simulink library "lpr"  (Simulink 8.1)
settings: Solver=ode1  StartTime=0.0  StopTime=Inf  FixedStep=0.001  RelTol=1e-3
PostLoadFcn:
  | , if any(exist('dsrtsu_mdlpostloadfcn', 'file') == [2, 3, 6]), try dsrtsu_mdlpostloadfcn('Execute', bdroot); catch fprintf('Error in PostLoadFcn (dsrtsu_mdlpostloadfcn) for model "%s":\n %s\n', bdroot, lasterr); end, end,
undefined symbols (not defined in the file or in its folder): ENUM_LANEQUALITY_MEDIUM, FALSE, KAPP_VehicleWidth_m, KPER_C0CrossingThr_m, KPER_CalDefaultTLC_s, KPER_CalTLCMax_s, KPER_CalTLCMin_s, KPER_DefaultLaneWidth_m, KPER_LaneWidHoldOnTime_s, KPER_LaneWidRampFinErrThres_m, KPER_LaneWidRampFinTimeThres_s, KPER_LaneWidRampInFalRt_mps, KPER_LaneWidRampInRisRt_mps, KPER_LaneWidRampOutFalRt_mps, KPER_LaneWidRampOutRisRt_mps, KPER_TLCDefaultValue_s, KPER_UseCalTLC_flg, TRUE
libraries: hcu_lib x6
settings Model: DSRTSU_INTERNAL_RTI_VER=450  DSRTSU_INTERNAL_RTI_TYPE=rti1401  RTICANMMDATA=struct('GeneralSetupData',struct('modelroot','D:\ELN150201_TAIWAN\trunk\AdasDragon\software\sw_development\arch\app\per','generalsettings',struct('filesettings',struct('destfolder',struct('Name','RTICANMM_FILES','Check',1),'buildfolder',struct('Name','.','Check',1),'AbsDestfolder',struct('Name','D:\ELN150201_TAIWAN\trunk\AdasDragon\software\sw_development\arch\app\per\RTICANMM_FILES'),'AbsBuildfolder',struct('Name','D:\ELN150201_TAIWAN\trunk\AdasDragon\software\sw_development\arch\app\per'))),'options',struct('addpaths',1,'rmpaths',1,'addtrcexclusion',logical(1),'cannavigator',struct('checkmonitoring',0),'show_usrtrc',0,'use_usrtrc',0),'advanced',struct('options',[1 1 1 1 1 1 1 1 1 1 1 1 1 1 1 1 1 1 1 1 1 1 1 1 1 1 1 1 1 1 1 1 1 1 1 1 1 1 1 1 1 1 1 1 1 1 1 1 1 1 1 1 1 1 1 1 1 1 1 1 1 1 1 1 1 1 1 1 1 1 1 1 1 1 1 1 1 1 1 1 1 1 1 1 1 1 1 1 1 1 1 1 1 1 1 1 1 1 1 1]),'MPSetup',{{}},'modelname','lpr','block','lpr'))  DSRTSU_INTERNAL_RTIFPGA=40  Creator=tescamilla  LastModifiedBy=AT015555

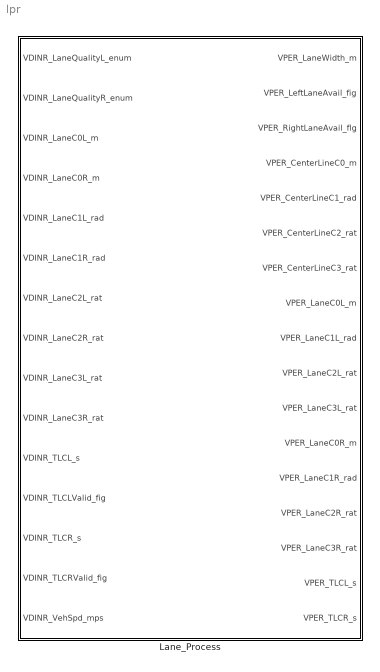
== system lpr ==
  Lane_Process : Subsystem  TreatAsAtomicUnit=on

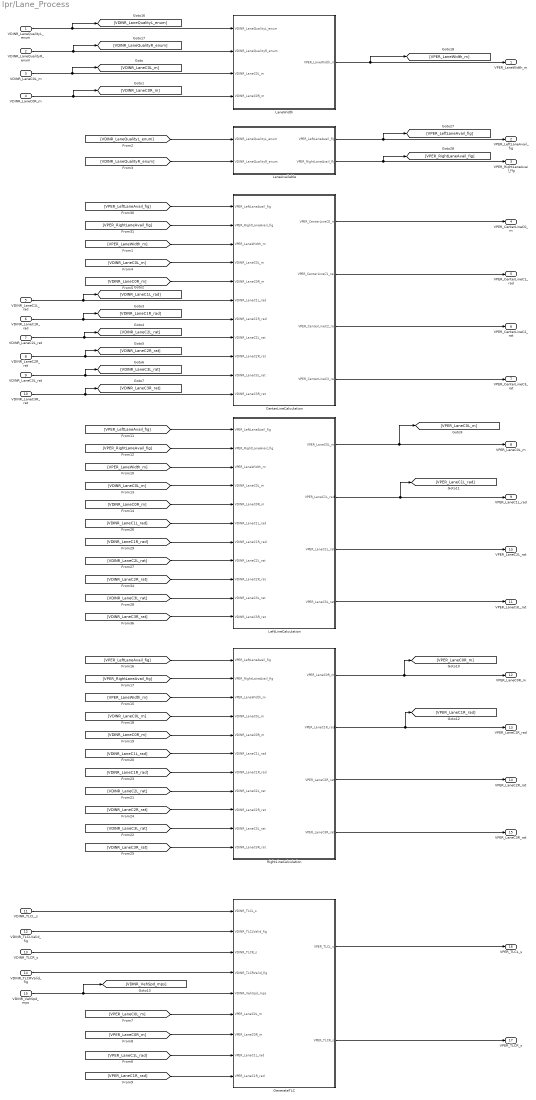
== system lpr/Lane_Process ==
  VDINR_LaneQualityL_enum : Inport
  VDINR_LaneQualityR_enum : Inport  Port=2
  VDINR_LaneC0L_m : Inport  Port=3
  VDINR_LaneC0R_m : Inport  Port=4
  VDINR_LaneC1L_rad : Inport  Port=5
  VDINR_LaneC1R_rad : Inport  Port=6
  VDINR_LaneC2L_rat : Inport  Port=7
  VDINR_LaneC2R_rat : Inport  Port=8
  VDINR_LaneC3L_rat : Inport  Port=9
  VDINR_LaneC3R_rat : Inport  Port=10
  VDINR_TLCL_s : Inport  Port=11
  VDINR_TLCLValid_fig : Inport  Port=12
  VDINR_TLCR_s : Inport  Port=13
  VDINR_TLCRValid_fig : Inport  Port=14
  VDINR_VehSpd_mps : Inport  Port=15
  CenterLineCalculation : Subsystem
  GenerateTLC : Subsystem
  LaneAvailable : Subsystem
  LaneWidth : Subsystem
  LeftLineCalculation : Subsystem
  RightLineCalculation : Subsystem
  VPER_LaneWidth_m : Outport
  VPER_LeftLaneAvail_fig : Outport  Port=2
  VPER_RightLaneAvail_flg : Outport  Port=3
  "VPER_CenterLineC0_m " : Outport  Port=4
  VPER_CenterLineC1_rad : Outport  Port=5
  VPER_CenterLineC2_rat : Outport  Port=6
  VPER_CenterLineC3_rat : Outport  Port=7
  VPER_LaneC0L_m : Outport  Port=8
  VPER_LaneC1L_rad : Outport  Port=9
  VPER_LaneC2L_rat : Outport  Port=10
  VPER_LaneC3L_rat : Outport  Port=11
  VPER_LaneC0R_m : Outport  Port=12
  VPER_LaneC1R_rad : Outport  Port=13
  VPER_LaneC2R_rat : Outport  Port=14
  VPER_LaneC3R_rat : Outport  Port=15
  VPER_TLCL_s : Outport  Port=16
  VPER_TLCR_s : Outport  Port=17
  wires:
  VDINR_LaneC1L_rad/1 -> CenterLineCalculation/6(VDINR_LaneC1L_rad), [VDINR_LaneC1L_rad]
  VDINR_LaneC1R_rad/1 -> CenterLineCalculation/7(VDINR_LaneC1R_rad), [VDINR_LaneC1R_rad]
  VDINR_LaneC2L_rat/1 -> CenterLineCalculation/8(VDINR_LaneC2L_rat), [VDINR_LaneC2L_rat]
  VDINR_LaneC2R_rat/1 -> CenterLineCalculation/9(VDINR_LaneC2R_rat), [VDINR_LaneC2R_rat]
  VDINR_LaneC3L_rat/1 -> CenterLineCalculation/10(VDINR_LaneC3L_rat), [VDINR_LaneC3L_rat]
  VDINR_LaneC3R_rat/1 -> CenterLineCalculation/11(VDINR_LaneC3R_rat), [VDINR_LaneC3R_rat]
  VDINR_LaneQualityL_enum/1 -> [VDINR_LaneQualityL_enum], LaneWidth/1(VDINR_LaneQualityL_enum)
  VDINR_LaneQualityR_enum/1 -> [VDINR_LaneQualityR_enum], LaneWidth/2(VDINR_LaneQualityR_enum)
  VDINR_LaneC0L_m/1 -> [VDINR_LaneC0L_m], LaneWidth/3(VDINR_LaneC0L_m)
  VDINR_LaneC0R_m/1 -> [VDINR_LaneC0R_m], LaneWidth/4(VDINR_LaneC0R_m)
  LaneWidth/1(VPER_LaneWidth_m) -> VPER_LaneWidth_m/1, [VPER_LaneWidth_m]
  LaneAvailable/2(VPER_RightLaneAvail_flg) -> [VPER_RightLaneAvail_fig], VPER_RightLaneAvail_flg/1
  LaneAvailable/1(VPER_LeftLaneAvail_flg) -> [VPER_LeftLaneAvail_fig], VPER_LeftLaneAvail_fig/1
  [VDINR_LaneQualityL_enum] -> LaneAvailable/1(VDINR_LaneQualityL_enum)
  [VDINR_LaneQualityR_enum] -> LaneAvailable/2(VDINR_LaneQualityR_enum)
  [VPER_LeftLaneAvail_fig] -> CenterLineCalculation/1(VPER_LeftLaneAvail_fig)
  [VPER_RightLaneAvail_fig] -> CenterLineCalculation/2(VPER_RightLaneAvail_fig)
  CenterLineCalculation/1("VPER_CenterLineC0_m ") -> "VPER_CenterLineC0_m "/1
  CenterLineCalculation/2(VPER_CenterLineC1_rad) -> VPER_CenterLineC1_rad/1
  CenterLineCalculation/3(VPER_CenterLineC2_rat) -> VPER_CenterLineC2_rat/1
  CenterLineCalculation/4(VPER_CenterLineC3_rat) -> VPER_CenterLineC3_rat/1
  VDINR_TLCL_s/1 -> GenerateTLC/1(VDINR_TLCL_s)
  VDINR_TLCLValid_fig/1 -> GenerateTLC/2(VDINR_TLCLValid_fig)
  VDINR_TLCR_s/1 -> GenerateTLC/3(VDINR_TLCR_s)
  VDINR_TLCRValid_fig/1 -> GenerateTLC/4(VDINR_TLCRValid_fig)
  GenerateTLC/1(VPER_TLCL_s) -> VPER_TLCL_s/1
  GenerateTLC/2(VPER_TLCR_s) -> VPER_TLCR_s/1
  [VPER_LaneWidth_m] -> CenterLineCalculation/3(VPER_LaneWidth_m)
  [VDINR_LaneC0L_m] -> CenterLineCalculation/4(VDINR_LaneC0L_m)
  [VDINR_LaneC0R_m] -> CenterLineCalculation/5(VDINR_LaneC0R_m)
  [VPER_LaneC1L_rad] -> GenerateTLC/8(VPER_LaneC1L_rad)
  [VPER_LaneC0L_m] -> GenerateTLC/6(VPER_LaneC0L_m)
  [VPER_LaneC0R_m] -> GenerateTLC/7(VPER_LaneC0R_m)
  VDINR_VehSpd_mps/1 -> [VDINR_VehSpd_mps], GenerateTLC/5(VDINR_VehSpd_mps)
  [VPER_LaneC1R_rad] -> GenerateTLC/9(VPER_LaneC1R_rad)
  [VDINR_LaneC0L_m] -> LeftLineCalculation/4(VDINR_LaneC0L_m)
  [VDINR_LaneC0R_m] -> LeftLineCalculation/5(VDINR_LaneC0R_m)
  [VPER_LaneWidth_m] -> LeftLineCalculation/3(VPER_LaneWidth_m)
  [VPER_RightLaneAvail_fig] -> LeftLineCalculation/2(VPER_RightLaneAvail_fig)
  [VPER_LeftLaneAvail_fig] -> LeftLineCalculation/1(VPER_LeftLaneAvail_fig)
  [VDINR_LaneC0L_m] -> RightLineCalculation/4(VDINR_LaneC0L_m)
  [VDINR_LaneC0R_m] -> RightLineCalculation/5(VDINR_LaneC0R_m)
  [VPER_LaneWidth_m] -> RightLineCalculation/3(VPER_LaneWidth_m)
  [VPER_RightLaneAvail_fig] -> RightLineCalculation/2(VPER_RightLaneAvail_fig)
  [VPER_LeftLaneAvail_fig] -> RightLineCalculation/1(VPER_LeftLaneAvail_fig)
  [VDINR_LaneC1L_rad] -> RightLineCalculation/6(VDINR_LaneC1L_rad)
  [VDINR_LaneC2L_rat] -> RightLineCalculation/8(VDINR_LaneC2L_rat)
  [VDINR_LaneC3L_rat] -> RightLineCalculation/10(VDINR_LaneC3L_rat)
  [VDINR_LaneC2R_rat] -> RightLineCalculation/9(VDINR_LaneC2R_rat)
  [VDINR_LaneC3R_rat] -> RightLineCalculation/11(VDINR_LaneC3R_rat)
  [VDINR_LaneC1R_rad] -> RightLineCalculation/7(VDINR_LaneC1R_rad)
  [VDINR_LaneC2L_rat] -> LeftLineCalculation/8(VDINR_LaneC2L_rat)
  [VDINR_LaneC2R_rat] -> LeftLineCalculation/9(VDINR_LaneC2R_rat)
  [VDINR_LaneC1L_rad] -> LeftLineCalculation/6(VDINR_LaneC1L_rad)
  [VDINR_LaneC3R_rat] -> LeftLineCalculation/11(VDINR_LaneC3R_rat)
  [VDINR_LaneC3L_rat] -> LeftLineCalculation/10(VDINR_LaneC3L_rat)
  [VDINR_LaneC1R_rad] -> LeftLineCalculation/7(VDINR_LaneC1R_rad)
  LeftLineCalculation/1(VPER_LaneC0L_m) -> VPER_LaneC0L_m/1, [VPER_LaneC0L_m]
  LeftLineCalculation/2(VPER_LaneC1L_rad) -> VPER_LaneC1L_rad/1, [VPER_LaneC1L_rad]
  LeftLineCalculation/3(VPER_LaneC2L_rat) -> VPER_LaneC2L_rat/1
  LeftLineCalculation/4(VPER_LaneC3L_rat) -> VPER_LaneC3L_rat/1
  RightLineCalculation/1(VPER_LaneC0R_m) -> VPER_LaneC0R_m/1, [VPER_LaneC0R_m]
  RightLineCalculation/2(VPER_LaneC1R_rad) -> VPER_LaneC1R_rad/1, [VPER_LaneC1R_rad]
  RightLineCalculation/3(VPER_LaneC2R_rat) -> VPER_LaneC2R_rat/1
  RightLineCalculation/4(VPER_LaneC3R_rat) -> VPER_LaneC3R_rat/1

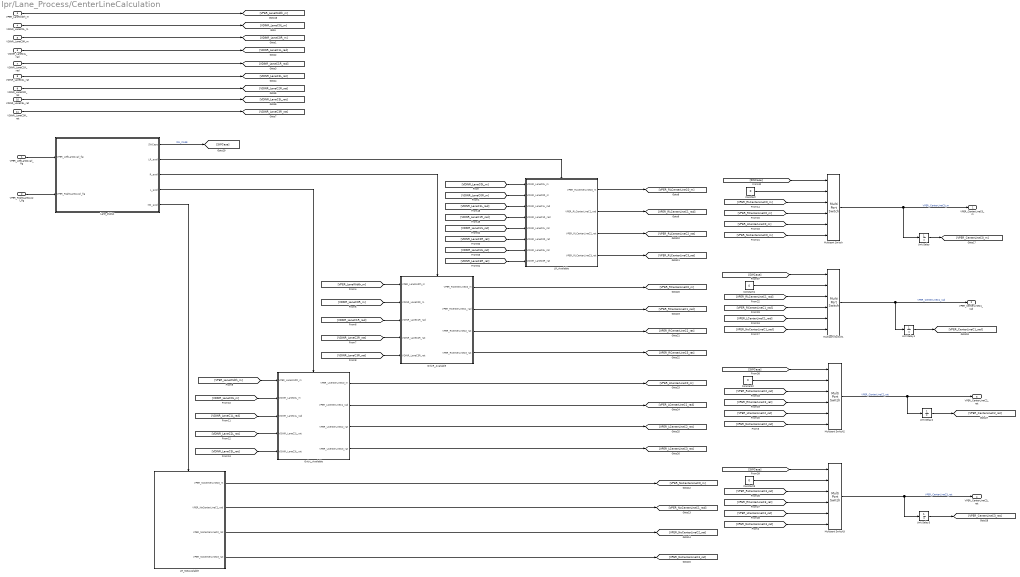
== system lpr/Lane_Process/CenterLineCalculation ==
  VPER_LeftLaneAvail_fig : Inport
  VPER_RightLaneAvail_fig : Inport  Port=2
  VPER_LaneWidth_m : Inport  Port=3
  VDINR_LaneC0L_m : Inport  Port=4
  VDINR_LaneC0R_m : Inport  Port=5
  VDINR_LaneC1L_rad : Inport  Port=6
  VDINR_LaneC1R_rad : Inport  Port=7
  VDINR_LaneC2L_rat : Inport  Port=8
  VDINR_LaneC2R_rat : Inport  Port=9
  VDINR_LaneC3L_rat : Inport  Port=10
  VDINR_LaneC3R_rat : Inport  Port=11
  Constant{,1..3} (4 alike) : Constant  Value=0  OutDataTypeStr=single
  LR_Available : Subsystem  TreatAsAtomicUnit=on
  LR_NotAvailable : Subsystem  TreatAsAtomicUnit=on
  Lane_status : Stateflow chart  TreatAsAtomicUnit=on
  Multiport Switch{,1..3} (4 alike) : MultiPortSwitch  DataPortOrder=Zero-based contiguous  Inputs=5
  OnlyL_Available : Subsystem  TreatAsAtomicUnit=on
  OnlyR_Available : Subsystem  TreatAsAtomicUnit=on
  Unit Delay{,1..3} (4 alike) : UnitDelay  SampleTime=-1
  "VPER_CenterLineC0_m " : Outport
  VPER_CenterLineC1_rad : Outport  Port=2
  VPER_CenterLineC2_rat : Outport  Port=3
  VPER_CenterLineC3_rat : Outport  Port=4
  wires:
  [VDINR_LaneC0R_m] -> LR_Available/2(VDINR_LaneC0R_m)
  [VDINR_LaneC0L_m] -> LR_Available/1(VDINR_LaneC0L_m)
  [VDINR_LaneC2L_rat] -> OnlyL_Available/4(VDINR_LaneC2L_rat)
  OnlyL_Available/1(VPER_LCenterLineC0_m) -> [VPER_LCenterLineC0_m]
  [VDINR_LaneC3L_rat] -> OnlyL_Available/5(VDINR_LaneC3L_rat)
  LR_Available/1(VPER_RLCenterLineC0_m) -> [VPER_RLCenterLineC0_m]
  OnlyR_Available/1(VPER_RCenterLineC0_m) -> [VPER_RCenterLineC0_m]
  LR_Available/2(VPER_RLCenterLineC1_rad) -> [VPER_RLCenterLineC1_rad]
  OnlyR_Available/2(VPER_RCenterLineC1_rad) -> [VPER_RCenterLineC1_rad]
  [VPER_LaneWidth_m] -> OnlyL_Available/1(VPER_LaneWidth_m)
  OnlyR_Available/3(VPER_RCenterLineC2_rat) -> [VPER_RCenterLineC2_rat]
  OnlyR_Available/4(VPER_RCenterLineC3_rat) -> [VPER_RCenterLineC3_rat]
  [VPER_LaneWidth_m] -> OnlyR_Available/1(VPER_LaneWidth_m)
  LR_Available/3(VPER_RLCenterLineC2_rat) -> [VPER_RLCenterLineC2_rat]
  LR_Available/4(VPER_RLCenterLineC3_rat) -> [VPER_RLCenterLineC3_rat]
  [VDINR_LaneC0R_m] -> OnlyR_Available/2(VDINR_LaneC0R_m)
  [VDINR_LaneC0L_m] -> OnlyL_Available/2(VDINR_LaneC0L_m)
  LR_NotAvailable/4(VPER_NoCenterLineC3_rat) -> [VPER_NoCenterLineC3_rat]
  LR_NotAvailable/1(VPER_NoCenterLineC0_m) -> [VPER_NoCenterLineC0_m]
  [VDINR_LaneC1R_rad] -> OnlyR_Available/3(VDINR_LaneC1R_rad)
  [VDINR_LaneC2R_rat] -> OnlyR_Available/4(VDINR_LaneC2R_rat)
  [VDINR_LaneC3R_rat] -> OnlyR_Available/5(VDINR_LaneC3R_rat)
  OnlyL_Available/4(VPER_LCenterLineC3_rat) -> [VPER_LCenterLineC3_rat]
  OnlyL_Available/3(VPER_LCenterLineC2_rat) -> [VPER_LCenterLineC2_rat]
  OnlyL_Available/2(VPER_LCenterLineC1_rad) -> [VPER_LCenterLineC1_rad]
  LR_NotAvailable/3(VPER_NoCenterLineC2_rat) -> [VPER_NoCenterLineC2_rat]
  LR_NotAvailable/2(VPER_NoCenterLineC1_rad) -> [VPER_NoCenterLineC1_rad]
  [VDINR_LaneC1L_rad] -> OnlyL_Available/3(VDINR_LaneC1L_rad)
  [VDINR_LaneC3R_rat] -> LR_Available/8(VDINR_LaneC3R_rat)
  [VDINR_LaneC3L_rat] -> LR_Available/7(VDINR_LaneC3L_rat)
  [VDINR_LaneC2L_rat] -> LR_Available/5(VDINR_LaneC2L_rat)
  [VDINR_LaneC1R_rad] -> LR_Available/4(VDINR_LaneC1R_rad)
  [VDINR_LaneC1L_rad] -> LR_Available/3(VDINR_LaneC1L_rad)
  [VDINR_LaneC2R_rat] -> LR_Available/6(VDINR_LaneC2R_rat)
  VDINR_LaneC0L_m/1 -> [VDINR_LaneC0L_m]
  VDINR_LaneC0R_m/1 -> [VDINR_LaneC0R_m]
  VDINR_LaneC1L_rad/1 -> [VDINR_LaneC1L_rad]
  VDINR_LaneC1R_rad/1 -> [VDINR_LaneC1R_rad]
  VDINR_LaneC2L_rat/1 -> [VDINR_LaneC2L_rat]
  VDINR_LaneC2R_rat/1 -> [VDINR_LaneC2R_rat]
  VDINR_LaneC3L_rat/1 -> [VDINR_LaneC3L_rat]
  VDINR_LaneC3R_rat/1 -> [VDINR_LaneC3R_rat]
  VPER_LaneWidth_m/1 -> [VPER_LaneWidth_m]
  Multiport Switch/1 -> Unit Delay/1, "VPER_CenterLineC0_m "/1  "VPER_CenterLineC0_m"
  Multiport Switch1/1 -> Unit Delay1/1, VPER_CenterLineC1_rad/1  "VPER_CenterLineC1_rad"
  Multiport Switch2/1 -> Unit Delay2/1, VPER_CenterLineC2_rat/1  "VPER_CenterLineC2_rat"
  Multiport Switch3/1 -> VPER_CenterLineC3_rat/1, Unit Delay3/1  "VPER_CenterLineC3_rat"
  Unit Delay/1 -> [VPER_CenterLineC0_m]
  Unit Delay1/1 -> [VPER_CenterLineC1_rad]
  Unit Delay2/1 -> [VPER_CenterLineC2_rat]
  Unit Delay3/1 -> [VPER_CenterLineC3_rat]
  VPER_LeftLaneAvail_fig/1 -> Lane_status/1(VPER_LeftLaneAvail_fig)
  VPER_RightLaneAvail_fig/1 -> Lane_status/2(VPER_RightLaneAvail_fig)
  Lane_status/1(SWCase) -> [SWCase]  "SW_CASE"
  Lane_status/2(LR_avail) -> LR_Available/Enable
  Lane_status/4(L_avail) -> OnlyL_Available/Enable
  Lane_status/3(R_avail) -> OnlyR_Available/Enable
  Lane_status/5(NO_avail) -> LR_NotAvailable/Enable
  [SWCase] -> Multiport Switch/1
  [VPER_RLCenterLineC0_m] -> Multiport Switch/3
  [VPER_RCenterLineC0_m] -> Multiport Switch/4
  [VPER_LCenterLineC0_m] -> Multiport Switch/5
  Constant/1 -> Multiport Switch/2
  [SWCase] -> Multiport Switch1/1
  [VPER_RLCenterLineC1_rad] -> Multiport Switch1/3
  [VPER_RCenterLineC1_rad] -> Multiport Switch1/4
  [VPER_LCenterLineC1_rad] -> Multiport Switch1/5
  Constant1/1 -> Multiport Switch1/2
  [SWCase] -> Multiport Switch2/1
  Constant2/1 -> Multiport Switch2/2
  [VPER_RLCenterLineC2_rat] -> Multiport Switch2/3
  [VPER_RCenterLineC2_rat] -> Multiport Switch2/4
  [VPER_LCenterLineC2_rat] -> Multiport Switch2/5
  [SWCase] -> Multiport Switch3/1
  Constant3/1 -> Multiport Switch3/2
  [VPER_RLCenterLineC3_rat] -> Multiport Switch3/3
  [VPER_RCenterLineC3_rat] -> Multiport Switch3/4
  [VPER_LCenterLineC3_rat] -> Multiport Switch3/5
  [VPER_NoCenterLineC3_rat] -> Multiport Switch3/6
  [VPER_NoCenterLineC2_rat] -> Multiport Switch2/6
  [VPER_NoCenterLineC1_rad] -> Multiport Switch1/6
  [VPER_NoCenterLineC0_m] -> Multiport Switch/6

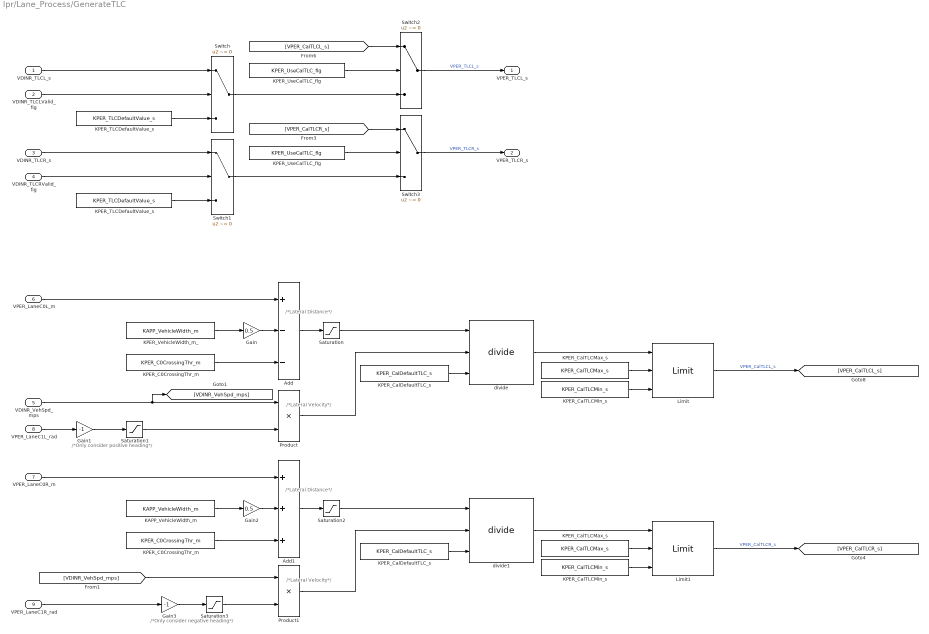
== system lpr/Lane_Process/GenerateTLC ==
  note: /*Lateral Velocity*/
  note: /*Lateral Distance*/
  note: /*Only consider positive heading*/
  note: /*Only consider negative heading*/
  note: /*Lateral Distance*/
  note: /*Lateral Velocity*/
  VDINR_TLCL_s : Inport
  VDINR_TLCLValid_fig : Inport  Port=2
  VDINR_TLCR_s : Inport  Port=3
  VDINR_TLCRValid_fig : Inport  Port=4
  VDINR_VehSpd_mps : Inport  Port=5
  VPER_LaneC0L_m : Inport  Port=6
  VPER_LaneC0R_m : Inport  Port=7
  VPER_LaneC1L_rad : Inport  Port=8
  VPER_LaneC1R_rad : Inport  Port=9
  Add : Sum  Inputs=+--
  Add1 : Sum  Inputs=+++
  Gain : Gain  Gain=0.5
  Gain1 : Gain  Gain=-1
  Gain2 : Gain  Gain=0.5
  Gain3 : Gain  Gain=-1
  "KAPP_VehicleWidth_m " : Constant  Value=KAPP_VehicleWidth_m
  KPER_C0CrossingThr_m : Constant  Value=KPER_C0CrossingThr_m
  "KPER_C0CrossingThr_m " : Constant  Value=KPER_C0CrossingThr_m
  KPER_CalDefaultTLC_s : Constant  Value=KPER_CalDefaultTLC_s
  "KPER_CalDefaultTLC_s " : Constant  Value=KPER_CalDefaultTLC_s
  KPER_CalTLCMax_s : Constant  Value=KPER_CalTLCMax_s
  "KPER_CalTLCMax_s " : Constant  Value=KPER_CalTLCMax_s
  KPER_CalTLCMin_s : Constant  Value=KPER_CalTLCMin_s
  "KPER_CalTLCMin_s " : Constant  Value=KPER_CalTLCMin_s
  KPER_TLCDefaultValue_s : Constant  Value=KPER_TLCDefaultValue_s
  "KPER_TLCDefaultValue_s " : Constant  Value=KPER_TLCDefaultValue_s
  KPER_UseCalTLC_flg : Constant  Value=KPER_UseCalTLC_flg
  "KPER_UseCalTLC_flg " : Constant  Value=KPER_UseCalTLC_flg
  KPER_VehicleWidth_m_ : Constant  Value=KAPP_VehicleWidth_m
  Limit : hcu_lib/Limit  SystemSampleTime=-1
  Limit1 : hcu_lib/Limit  SystemSampleTime=-1
  Product : Product
  Product1 : Product
  Saturation : Saturate  UpperLimit=inf  LowerLimit=0
  Saturation1 : Saturate  UpperLimit=inf  LowerLimit=0
  Saturation2 : Saturate  UpperLimit=0  LowerLimit=-inf
  Saturation3 : Saturate  UpperLimit=0  LowerLimit=-inf
  Switch{,1..3} (4 alike) : Switch  Criteria=u2 ~= 0
  divide : hcu_lib/divide
  divide1 : hcu_lib/divide
  VPER_TLCL_s : Outport
  VPER_TLCR_s : Outport  Port=2
  wires:
  VDINR_TLCRValid_fig/1 -> Switch1/2
  Switch3/1 -> VPER_TLCR_s/1  "VPER_TLCR_s"
  "KPER_TLCDefaultValue_s "/1 -> Switch1/3
  Switch2/1 -> VPER_TLCL_s/1  "VPER_TLCL_s"
  KPER_TLCDefaultValue_s/1 -> Switch/3
  VDINR_TLCLValid_fig/1 -> Switch/2
  Gain/1 -> Add/2
  VPER_LaneC0L_m/1 -> Add/1
  KPER_VehicleWidth_m_/1 -> Gain/1
  KPER_C0CrossingThr_m/1 -> Add/3
  VDINR_VehSpd_mps/1 -> Product/1, [VDINR_VehSpd_mps]
  VPER_LaneC1L_rad/1 -> Gain1/1
  Product/1 -> divide/2
  Add/1 -> Saturation/1
  KPER_CalDefaultTLC_s/1 -> divide/3
  Saturation/1 -> divide/1
  Saturation1/1 -> Product/2
  Gain1/1 -> Saturation1/1
  divide/1 -> Limit/1
  KPER_CalTLCMax_s/1 -> Limit/2
  KPER_CalTLCMin_s/1 -> Limit/3
  Limit/1 -> [VPER_CalTLCL_s]  "VPER_CalTLCL_s"
  Saturation3/1 -> Product1/2
  Saturation2/1 -> divide1/1
  "KPER_CalDefaultTLC_s "/1 -> divide1/3
  Add1/1 -> Saturation2/1
  Product1/1 -> divide1/2
  [VDINR_VehSpd_mps] -> Product1/1
  "KPER_C0CrossingThr_m "/1 -> Add1/3
  "KAPP_VehicleWidth_m "/1 -> Gain2/1
  Gain2/1 -> Add1/2
  VPER_LaneC0R_m/1 -> Add1/1
  "KPER_CalTLCMax_s "/1 -> Limit1/2
  "KPER_CalTLCMin_s "/1 -> Limit1/3
  Limit1/1 -> [VPER_CalTLCR_s]  "VPER_CalTLCR_s"
  divide1/1 -> Limit1/1
  Gain3/1 -> Saturation3/1
  VPER_LaneC1R_rad/1 -> Gain3/1
  [VPER_CalTLCL_s] -> Switch2/1
  VDINR_TLCL_s/1 -> Switch/1
  VDINR_TLCR_s/1 -> Switch1/1
  [VPER_CalTLCR_s] -> Switch3/1
  KPER_UseCalTLC_flg/1 -> Switch2/2
  "KPER_UseCalTLC_flg "/1 -> Switch3/2
  Switch/1 -> Switch2/3
  Switch1/1 -> Switch3/3

== system lpr/Lane_Process/LaneAvailable ==
  VDINR_LaneQualityL_enum : Inport
  VDINR_LaneQualityR_enum : Inport  Port=2
  Constant2 : Constant  Value=ENUM_LANEQUALITY_MEDIUM
  Constant3 : Constant  Value=ENUM_LANEQUALITY_MEDIUM
  Relational Operator : RelationalOperator  OutDataTypeStr=boolean
  Relational Operator1 : RelationalOperator  OutDataTypeStr=boolean
  VPER_LeftLaneAvail_flg : Outport
  VPER_RightLaneAvail_flg : Outport  Port=2
  wires:
  Relational Operator1/1 -> VPER_RightLaneAvail_flg/1  "VPER_RightLaneAvail_flg"
  VDINR_LaneQualityR_enum/1 -> Relational Operator1/1
  Constant2/1 -> Relational Operator/2
  Constant3/1 -> Relational Operator1/2
  VDINR_LaneQualityL_enum/1 -> Relational Operator/1
  Relational Operator/1 -> VPER_LeftLaneAvail_flg/1  "VPER_LeftLaneAvail_flg"

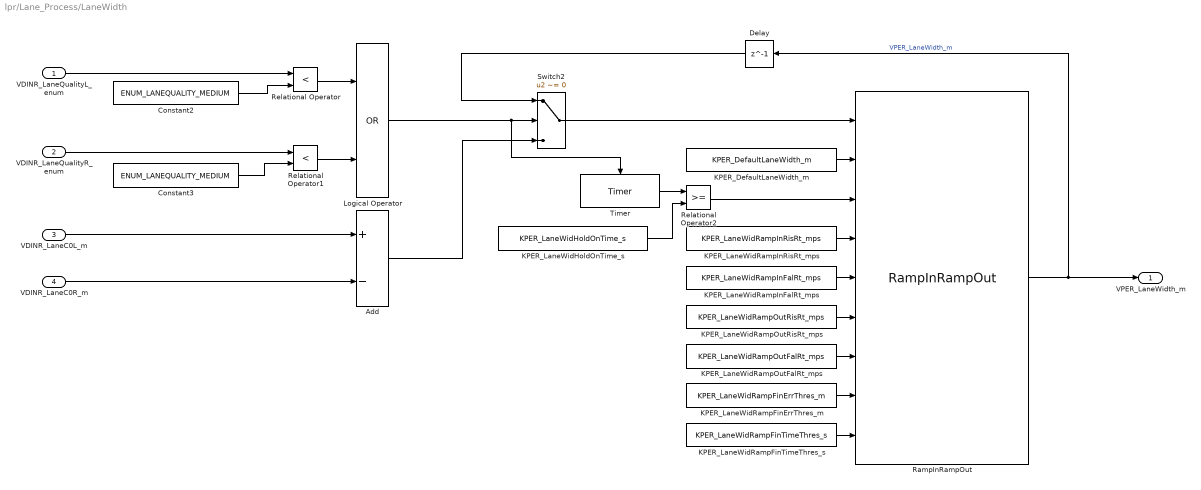
== system lpr/Lane_Process/LaneWidth ==
  VDINR_LaneQualityL_enum : Inport
  VDINR_LaneQualityR_enum : Inport  Port=2
  VDINR_LaneC0L_m : Inport  Port=3
  VDINR_LaneC0R_m : Inport  Port=4
  Add : Sum  Inputs=+-
  Constant2 : Constant  Value=ENUM_LANEQUALITY_MEDIUM
  Constant3 : Constant  Value=ENUM_LANEQUALITY_MEDIUM
  Delay : Delay  DelayLength=1  InitialCondition=KPER_DefaultLaneWidth_m
  KPER_DefaultLaneWidth_m : Constant  Value=KPER_DefaultLaneWidth_m
  KPER_LaneWidHoldOnTime_s : Constant  Value=KPER_LaneWidHoldOnTime_s
  KPER_LaneWidRampFinErrThres_m : Constant  Value=KPER_LaneWidRampFinErrThres_m
  KPER_LaneWidRampFinTimeThres_s : Constant  Value=KPER_LaneWidRampFinTimeThres_s
  KPER_LaneWidRampInFalRt_mps : Constant  Value=KPER_LaneWidRampInFalRt_mps
  KPER_LaneWidRampInRisRt_mps : Constant  Value=KPER_LaneWidRampInRisRt_mps
  KPER_LaneWidRampOutFalRt_mps : Constant  Value=KPER_LaneWidRampOutFalRt_mps
  KPER_LaneWidRampOutRisRt_mps : Constant  Value=KPER_LaneWidRampOutRisRt_mps
  Logical Operator : Logic  Operator=OR  AllPortsSameDT=off  OutDataTypeStr=boolean
  RampInRampOut : hcu_lib/RampInRampOut  SystemSampleTime=-1
  Relational Operator : RelationalOperator  Operator=<  OutDataTypeStr=boolean
  Relational Operator1 : RelationalOperator  Operator=<  OutDataTypeStr=boolean
  Relational Operator2 : RelationalOperator  OutDataTypeStr=boolean
  Switch2 : Switch  Criteria=u2 ~= 0
  Timer : hcu_lib/Timer  SystemSampleTime=-1
  VPER_LaneWidth_m : Outport
  wires:
  Constant2/1 -> Relational Operator/2
  Constant3/1 -> Relational Operator1/2
  VDINR_LaneQualityR_enum/1 -> Relational Operator1/1
  VDINR_LaneQualityL_enum/1 -> Relational Operator/1
  VDINR_LaneC0R_m/1 -> Add/2
  Add/1 -> Switch2/3
  VDINR_LaneC0L_m/1 -> Add/1
  Relational Operator1/1 -> Logical Operator/2
  Relational Operator/1 -> Logical Operator/1
  Switch2/1 -> RampInRampOut/1
  Delay/1 -> Switch2/1
  KPER_DefaultLaneWidth_m/1 -> RampInRampOut/2
  Logical Operator/1 -> Switch2/2, Timer/Enable
  KPER_LaneWidRampInRisRt_mps/1 -> RampInRampOut/4
  KPER_LaneWidRampInFalRt_mps/1 -> RampInRampOut/5
  KPER_LaneWidRampOutFalRt_mps/1 -> RampInRampOut/7
  KPER_LaneWidRampOutRisRt_mps/1 -> RampInRampOut/6
  KPER_LaneWidRampFinErrThres_m/1 -> RampInRampOut/8
  KPER_LaneWidRampFinTimeThres_s/1 -> RampInRampOut/9
  RampInRampOut/1 -> Delay/1, VPER_LaneWidth_m/1  "VPER_LaneWidth_m"
  Relational Operator2/1 -> RampInRampOut/3
  Timer/1 -> Relational Operator2/1
  KPER_LaneWidHoldOnTime_s/1 -> Relational Operator2/2

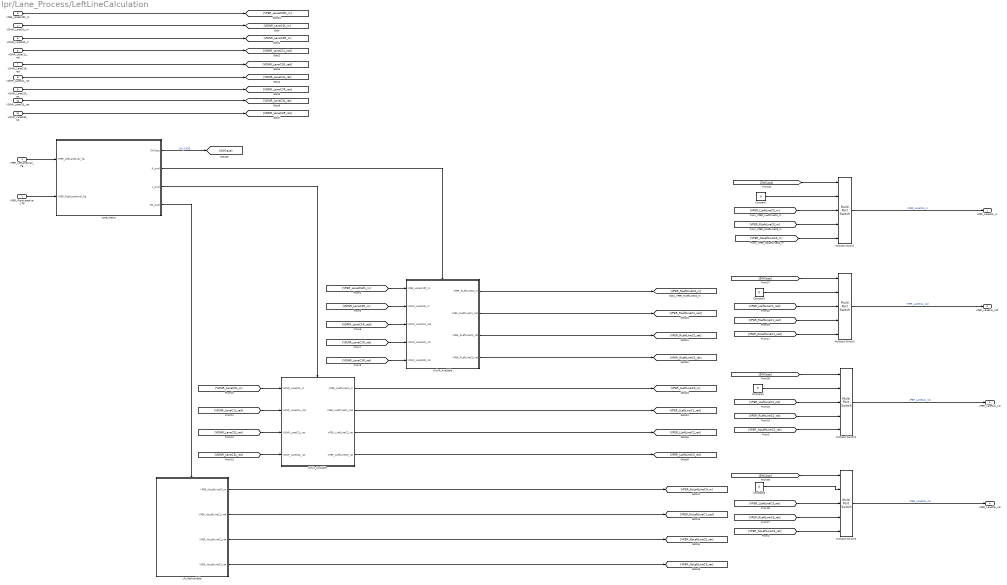
== system lpr/Lane_Process/LeftLineCalculation ==
  VPER_LeftLaneAvail_fig : Inport
  VPER_RightLaneAvail_fig : Inport  Port=2
  VPER_LaneWidth_m : Inport  Port=3
  VDINR_LaneC0L_m : Inport  Port=4
  VDINR_LaneC0R_m : Inport  Port=5
  VDINR_LaneC1L_rad : Inport  Port=6
  VDINR_LaneC1R_rad : Inport  Port=7
  VDINR_LaneC2L_rat : Inport  Port=8
  VDINR_LaneC2R_rat : Inport  Port=9
  VDINR_LaneC3L_rat : Inport  Port=10
  VDINR_LaneC3R_rat : Inport  Port=11
  Constant{,1..3} (4 alike) : Constant  Value=0  OutDataTypeStr=single
  LR_NotAvailable : Subsystem  TreatAsAtomicUnit=on
  Lane_status : Stateflow chart  TreatAsAtomicUnit=on
  Multiport Switch{,1..3} (4 alike) : MultiPortSwitch  DataPortOrder=Zero-based contiguous  Inputs=4
  OnlyL_Available : Subsystem  TreatAsAtomicUnit=on
  OnlyR_Available : Subsystem  TreatAsAtomicUnit=on
  VPER_LaneC0L_m : Outport
  VPER_LaneC1L_rad : Outport  Port=2
  VPER_LaneC2L_rat : Outport  Port=3
  VPER_LaneC3L_rat : Outport  Port=4
  wires:
  [VPER_NoLeftLineC0_m] -> Multiport Switch/5
  [VPER_NoLeftLineC1_rad] -> Multiport Switch1/5
  [VPER_NoLeftLineC2_rat] -> Multiport Switch2/5
  [VPER_NoLeftLineC3_rat] -> Multiport Switch3/5
  [VPER_LLeftLineC3_rat] -> Multiport Switch3/3
  [VPER_RLeftLineC3_rat] -> Multiport Switch3/4
  Constant3/1 -> Multiport Switch3/2
  [SWCase] -> Multiport Switch3/1
  [VPER_LLeftLineC2_rat] -> Multiport Switch2/3
  [VPER_RLeftLineC2_rat] -> Multiport Switch2/4
  Constant2/1 -> Multiport Switch2/2
  [SWCase] -> Multiport Switch2/1
  Constant1/1 -> Multiport Switch1/2
  [VPER_LLeftLineC1_rad] -> Multiport Switch1/3
  [VPER_RLeftLineC1_rad] -> Multiport Switch1/4
  [SWCase] -> Multiport Switch1/1
  Constant/1 -> Multiport Switch/2
  [VPER_LLeftLineC0_m] -> Multiport Switch/3
  [VPER_RLeftLineC0_m] -> Multiport Switch/4
  [SWCase] -> Multiport Switch/1
  Lane_status/4(NO_avail) -> LR_NotAvailable/Enable
  Lane_status/2(R_avail) -> OnlyR_Available/Enable
  Lane_status/3(L_avail) -> OnlyL_Available/Enable
  Lane_status/1(SWCase) -> [SWCase]  "SW_CASE"
  VPER_RightLaneAvail_fig/1 -> Lane_status/2(VPER_RightLaneAvail_fig)
  VPER_LeftLaneAvail_fig/1 -> Lane_status/1(VPER_LeftLaneAvail_fig)
  Multiport Switch3/1 -> VPER_LaneC3L_rat/1  "VPER_LaneC3L_rat"
  Multiport Switch2/1 -> VPER_LaneC2L_rat/1  "VPER_LaneC2L_rat"
  Multiport Switch1/1 -> VPER_LaneC1L_rad/1  "VPER_LaneC1L_rad"
  Multiport Switch/1 -> VPER_LaneC0L_m/1  "VPER_LaneC0L_m"
  VPER_LaneWidth_m/1 -> [VPER_LaneWidth_m]
  VDINR_LaneC3R_rat/1 -> [VDINR_LaneC3R_rat]
  VDINR_LaneC3L_rat/1 -> [VDINR_LaneC3L_rat]
  VDINR_LaneC2R_rat/1 -> [VDINR_LaneC2R_rat]
  VDINR_LaneC2L_rat/1 -> [VDINR_LaneC2L_rat]
  VDINR_LaneC1R_rad/1 -> [VDINR_LaneC1R_rad]
  VDINR_LaneC1L_rad/1 -> [VDINR_LaneC1L_rad]
  VDINR_LaneC0R_m/1 -> [VDINR_LaneC0R_m]
  VDINR_LaneC0L_m/1 -> [VDINR_LaneC0L_m]
  [VDINR_LaneC1L_rad] -> OnlyL_Available/2(VDINR_LaneC1L_rad)
  LR_NotAvailable/2(VPER_NoLeftLineC1_rad) -> [VPER_NoLeftLineC1_rad]
  LR_NotAvailable/3(VPER_NoLeftLineC2_rat) -> [VPER_NoLeftLineC2_rat]
  OnlyL_Available/2(VPER_LLeftLineC1_rad) -> [VPER_LLeftLineC1_rad]
  OnlyL_Available/3(VPER_LLeftLineC2_rat) -> [VPER_LLeftLineC2_rat]
  OnlyL_Available/4(VPER_LLeftLineC3_rat) -> [VPER_LLeftLineC3_rat]
  [VDINR_LaneC3R_rat] -> OnlyR_Available/5(VDINR_LaneC3R_rat)
  [VDINR_LaneC2R_rat] -> OnlyR_Available/4(VDINR_LaneC2R_rat)
  [VDINR_LaneC1R_rad] -> OnlyR_Available/3(VDINR_LaneC1R_rad)
  LR_NotAvailable/1(VPER_NoLeftLineC0_m) -> [VPER_NoLeftLineC0_m]
  LR_NotAvailable/4(VPER_NoLeftLineC3_rat) -> [VPER_NoLeftLineC3_rat]
  [VDINR_LaneC0L_m] -> OnlyL_Available/1(VDINR_LaneC0L_m)
  [VDINR_LaneC0R_m] -> OnlyR_Available/2(VDINR_LaneC0R_m)
  [VPER_LaneWidth_m] -> OnlyR_Available/1(VPER_LaneWidth_m)
  OnlyR_Available/4(VPER_RLeftLineC3_rat) -> [VPER_RLeftLineC3_rat]
  OnlyR_Available/3(VPER_RLeftLineC2_rat) -> [VPER_RLeftLineC2_rat]
  OnlyR_Available/2(VPER_RLeftLineC1_rad) -> [VPER_RLeftLineC1_rad]
  OnlyR_Available/1(VPER_RLeftLineC0_m) -> [VPER_RLeftLineC0_m]
  [VDINR_LaneC3L_rat] -> OnlyL_Available/4(VDINR_LaneC3L_rat)
  OnlyL_Available/1(VPER_LLeftLineC0_m) -> [VPER_LLeftLineC0_m]
  [VDINR_LaneC2L_rat] -> OnlyL_Available/3(VDINR_LaneC2L_rat)

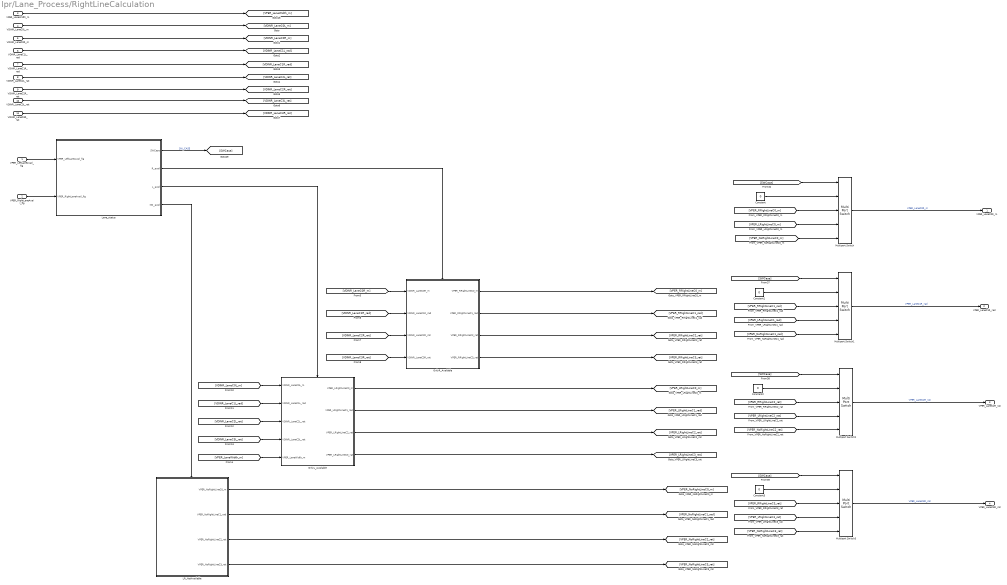
== system lpr/Lane_Process/RightLineCalculation ==
  VPER_LeftLaneAvail_fig : Inport
  VPER_RightLaneAvail_fig : Inport  Port=2
  VPER_LaneWidth_m : Inport  Port=3
  VDINR_LaneC0L_m : Inport  Port=4
  VDINR_LaneC0R_m : Inport  Port=5
  VDINR_LaneC1L_rad : Inport  Port=6
  VDINR_LaneC1R_rad : Inport  Port=7
  VDINR_LaneC2L_rat : Inport  Port=8
  VDINR_LaneC2R_rat : Inport  Port=9
  VDINR_LaneC3L_rat : Inport  Port=10
  VDINR_LaneC3R_rat : Inport  Port=11
  Constant{,1..3} (4 alike) : Constant  Value=0  OutDataTypeStr=single
  LR_NotAvailable : Subsystem  TreatAsAtomicUnit=on
  Lane_status : Stateflow chart  TreatAsAtomicUnit=on
  Multiport Switch{,1..3} (4 alike) : MultiPortSwitch  DataPortOrder=Zero-based contiguous  Inputs=4
  OnlyL_Available : Subsystem  TreatAsAtomicUnit=on
  OnlyR_Available : Subsystem  TreatAsAtomicUnit=on
  VPER_LaneC0R_m : Outport
  VPER_LaneC1R_rad : Outport  Port=2
  VPER_LaneC2R_rat : Outport  Port=3
  VPER_LaneC3R_rat : Outport  Port=4
  wires:
  [VDINR_LaneC2L_rat] -> OnlyL_Available/3(VDINR_LaneC2L_rat)
  OnlyL_Available/1(VPER_LRightLineC0_m) -> [VPER_LRightLineC0_m]
  [VDINR_LaneC3L_rat] -> OnlyL_Available/4(VDINR_LaneC3L_rat)
  OnlyR_Available/1(VPER_RRightLineC0_m) -> [VPER_RRightLineC0_m]
  OnlyR_Available/2(VPER_RRightLineC1_rad) -> [VPER_RRightLineC1_rad]
  OnlyR_Available/3(VPER_RRightLineC2_rat) -> [VPER_RRightLineC2_rat]
  OnlyR_Available/4(VPER_RRightLineC3_rat) -> [VPER_RRightLineC3_rat]
  [VDINR_LaneC0R_m] -> OnlyR_Available/1(VDINR_LaneC0R_m)
  [VDINR_LaneC0L_m] -> OnlyL_Available/1(VDINR_LaneC0L_m)
  LR_NotAvailable/4(VPER_NoRightLineC3_rat) -> [VPER_NoRightLineC3_rat]
  LR_NotAvailable/1(VPER_NoRightLineC0_m) -> [VPER_NoRightLineC0_m]
  [VDINR_LaneC1R_rad] -> OnlyR_Available/2(VDINR_LaneC1R_rad)
  [VDINR_LaneC2R_rat] -> OnlyR_Available/3(VDINR_LaneC2R_rat)
  [VDINR_LaneC3R_rat] -> OnlyR_Available/4(VDINR_LaneC3R_rat)
  OnlyL_Available/4(VPER_LRightLineC3_rat) -> [VPER_LRightLineC3_rat]
  OnlyL_Available/3(VPER_LRightLineC2_rat) -> [VPER_LRightLineC2_rat]
  OnlyL_Available/2(VPER_LRightLineC1_rad) -> [VPER_LRightLineC1_rad]
  LR_NotAvailable/3(VPER_NoRightLineC2_rat) -> [VPER_NoRightLineC2_rat]
  LR_NotAvailable/2(VPER_NoRightLineC1_rad) -> [VPER_NoRightLineC1_rad]
  [VDINR_LaneC1L_rad] -> OnlyL_Available/2(VDINR_LaneC1L_rad)
  VDINR_LaneC0L_m/1 -> [VDINR_LaneC0L_m]
  VDINR_LaneC0R_m/1 -> [VDINR_LaneC0R_m]
  VDINR_LaneC1L_rad/1 -> [VDINR_LaneC1L_rad]
  VDINR_LaneC1R_rad/1 -> [VDINR_LaneC1R_rad]
  VDINR_LaneC2L_rat/1 -> [VDINR_LaneC2L_rat]
  VDINR_LaneC2R_rat/1 -> [VDINR_LaneC2R_rat]
  VDINR_LaneC3L_rat/1 -> [VDINR_LaneC3L_rat]
  VDINR_LaneC3R_rat/1 -> [VDINR_LaneC3R_rat]
  VPER_LaneWidth_m/1 -> [VPER_LaneWidth_m]
  Multiport Switch/1 -> VPER_LaneC0R_m/1  "VPER_LaneC0R_m"
  Multiport Switch1/1 -> VPER_LaneC1R_rad/1  "VPER_LaneC1R_rad"
  Multiport Switch2/1 -> VPER_LaneC2R_rat/1  "VPER_LaneC2R_rat"
  Multiport Switch3/1 -> VPER_LaneC3R_rat/1  "VPER_LaneC3R_rat"
  VPER_LeftLaneAvail_fig/1 -> Lane_status/1(VPER_LeftLaneAvail_fig)
  VPER_RightLaneAvail_fig/1 -> Lane_status/2(VPER_RightLaneAvail_fig)
  Lane_status/1(SWCase) -> [SWCase]  "SW_CASE"
  Lane_status/3(L_avail) -> OnlyL_Available/Enable
  Lane_status/2(R_avail) -> OnlyR_Available/Enable
  Lane_status/4(NO_avail) -> LR_NotAvailable/Enable
  [SWCase] -> Multiport Switch/1
  [VPER_LRightLineC0_m] -> Multiport Switch/4
  [VPER_RRightLineC0_m] -> Multiport Switch/3
  Constant/1 -> Multiport Switch/2
  [SWCase] -> Multiport Switch1/1
  [VPER_RRightLineC1_rad] -> Multiport Switch1/3
  [VPER_LRightLineC1_rad] -> Multiport Switch1/4
  Constant1/1 -> Multiport Switch1/2
  [SWCase] -> Multiport Switch2/1
  Constant2/1 -> Multiport Switch2/2
  [VPER_LRightLineC2_rat] -> Multiport Switch2/4
  [VPER_RRightLineC2_rat] -> Multiport Switch2/3
  [SWCase] -> Multiport Switch3/1
  Constant3/1 -> Multiport Switch3/2
  [VPER_LRightLineC3_rat] -> Multiport Switch3/4
  [VPER_RRightLineC3_rat] -> Multiport Switch3/3
  [VPER_NoRightLineC3_rat] -> Multiport Switch3/5
  [VPER_NoRightLineC2_rat] -> Multiport Switch2/5
  [VPER_NoRightLineC1_rad] -> Multiport Switch1/5
  [VPER_NoRightLineC0_m] -> Multiport Switch/5
  [VPER_LaneWidth_m] -> OnlyL_Available/5(VPER_LaneWidth_m)

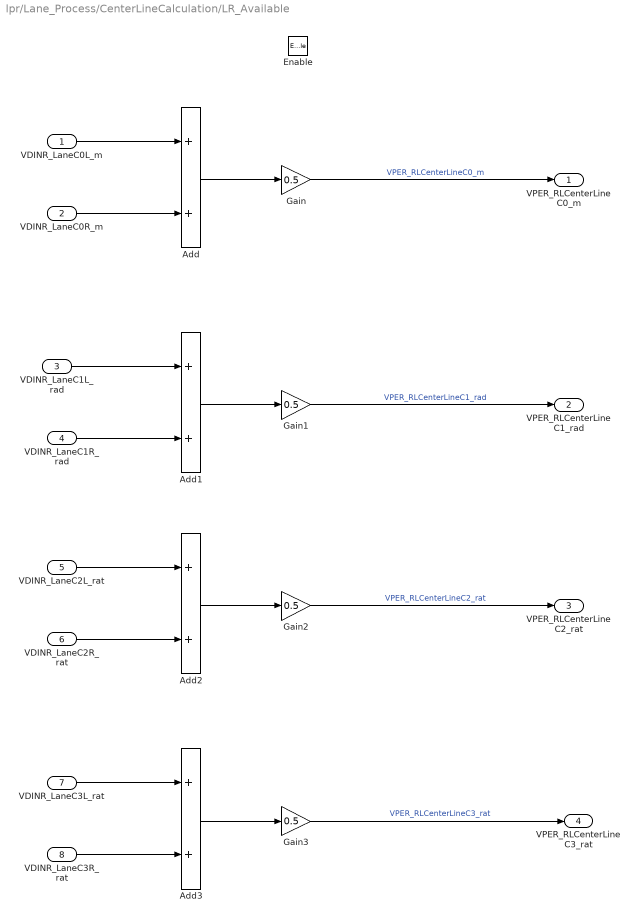
== system lpr/Lane_Process/CenterLineCalculation/LR_Available ==
  VDINR_LaneC0L_m : Inport
  VDINR_LaneC0R_m : Inport  Port=2
  VDINR_LaneC1L_rad : Inport  Port=3
  VDINR_LaneC1R_rad : Inport  Port=4
  VDINR_LaneC2L_rat : Inport  Port=5
  VDINR_LaneC2R_rat : Inport  Port=6
  VDINR_LaneC3L_rat : Inport  Port=7
  VDINR_LaneC3R_rat : Inport  Port=8
  Enable : EnablePort  StatesWhenEnabling=reset
  Add{,1..3} (4 alike) : Sum
  Gain{,1..3} (4 alike) : Gain  Gain=0.5
  VPER_RLCenterLineC0_m : Outport
  VPER_RLCenterLineC1_rad : Outport  Port=2
  VPER_RLCenterLineC2_rat : Outport  Port=3
  VPER_RLCenterLineC3_rat : Outport  Port=4
  wires:
  VDINR_LaneC0L_m/1 -> Add/1
  VDINR_LaneC0R_m/1 -> Add/2
  Add/1 -> Gain/1
  Gain/1 -> VPER_RLCenterLineC0_m/1  "VPER_RLCenterLineC0_m"
  VDINR_LaneC1L_rad/1 -> Add1/1
  VDINR_LaneC1R_rad/1 -> Add1/2
  Add1/1 -> Gain1/1
  Add2/1 -> Gain2/1
  Gain1/1 -> VPER_RLCenterLineC1_rad/1  "VPER_RLCenterLineC1_rad"
  VDINR_LaneC2L_rat/1 -> Add2/1
  VDINR_LaneC2R_rat/1 -> Add2/2
  Gain2/1 -> VPER_RLCenterLineC2_rat/1  "VPER_RLCenterLineC2_rat"
  Add3/1 -> Gain3/1
  VDINR_LaneC3L_rat/1 -> Add3/1
  VDINR_LaneC3R_rat/1 -> Add3/2
  Gain3/1 -> VPER_RLCenterLineC3_rat/1  "VPER_RLCenterLineC3_rat"

== system lpr/Lane_Process/CenterLineCalculation/LR_NotAvailable ==
  Enable : EnablePort  StatesWhenEnabling=reset
  Constant{,1..3} (4 alike) : Constant  Value=0  OutDataTypeStr=single
  VPER_NoCenterLineC0_m : Outport
  VPER_NoCenterLineC1_rad : Outport  Port=2
  VPER_NoCenterLineC2_rat : Outport  Port=3
  VPER_NoCenterLineC3_rat : Outport  Port=4
  wires:
  Constant/1 -> VPER_NoCenterLineC0_m/1
  Constant1/1 -> VPER_NoCenterLineC1_rad/1
  Constant2/1 -> VPER_NoCenterLineC2_rat/1
  Constant3/1 -> VPER_NoCenterLineC3_rat/1

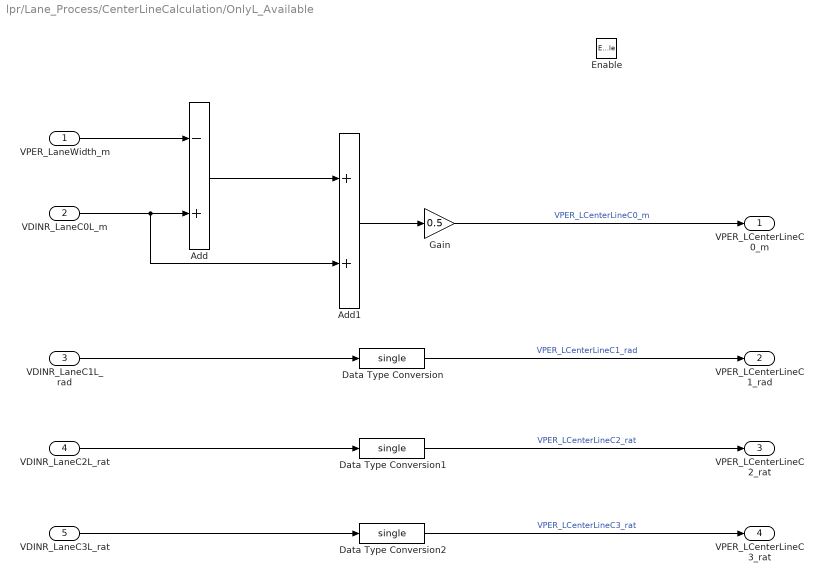
== system lpr/Lane_Process/CenterLineCalculation/OnlyL_Available ==
  VPER_LaneWidth_m : Inport
  VDINR_LaneC0L_m : Inport  Port=2
  VDINR_LaneC1L_rad : Inport  Port=3
  VDINR_LaneC2L_rat : Inport  Port=4
  VDINR_LaneC3L_rat : Inport  Port=5
  Enable : EnablePort  StatesWhenEnabling=reset
  Add : Sum  Inputs=-+
  Add1 : Sum
  Data Type Conversion : DataTypeConversion  OutDataTypeStr=single
  Data Type Conversion1 : DataTypeConversion  OutDataTypeStr=single
  Data Type Conversion2 : DataTypeConversion  OutDataTypeStr=single
  Gain : Gain  Gain=0.5
  VPER_LCenterLineC0_m : Outport
  VPER_LCenterLineC1_rad : Outport  Port=2
  VPER_LCenterLineC2_rat : Outport  Port=3
  VPER_LCenterLineC3_rat : Outport  Port=4
  wires:
  VDINR_LaneC1L_rad/1 -> Data Type Conversion/1
  VPER_LaneWidth_m/1 -> Add/1
  VDINR_LaneC0L_m/1 -> Add1/2, Add/2
  VDINR_LaneC2L_rat/1 -> Data Type Conversion1/1
  VDINR_LaneC3L_rat/1 -> Data Type Conversion2/1
  Add/1 -> Add1/1
  Add1/1 -> Gain/1
  Gain/1 -> VPER_LCenterLineC0_m/1  "VPER_LCenterLineC0_m"
  Data Type Conversion1/1 -> VPER_LCenterLineC2_rat/1  "VPER_LCenterLineC2_rat"
  Data Type Conversion2/1 -> VPER_LCenterLineC3_rat/1  "VPER_LCenterLineC3_rat"
  Data Type Conversion/1 -> VPER_LCenterLineC1_rad/1  "VPER_LCenterLineC1_rad"

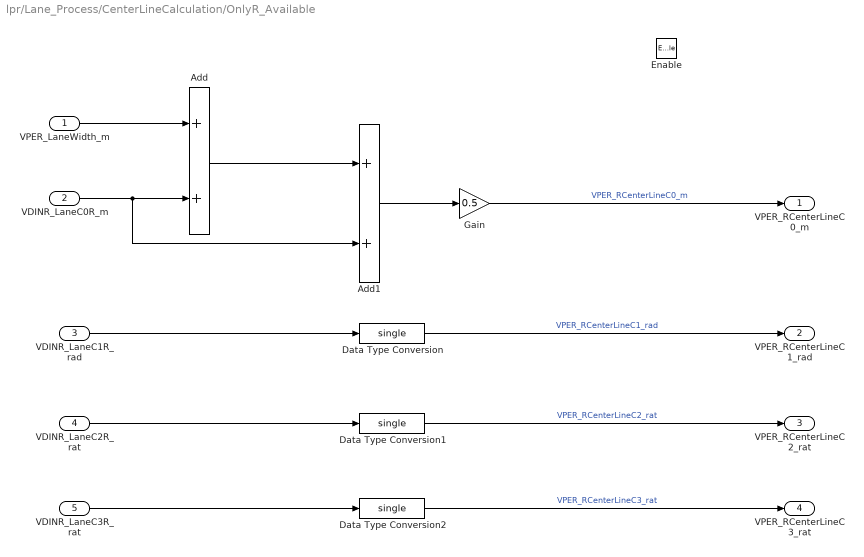
== system lpr/Lane_Process/CenterLineCalculation/OnlyR_Available ==
  VPER_LaneWidth_m : Inport
  VDINR_LaneC0R_m : Inport  Port=2
  VDINR_LaneC1R_rad : Inport  Port=3
  VDINR_LaneC2R_rat : Inport  Port=4
  VDINR_LaneC3R_rat : Inport  Port=5
  Enable : EnablePort  StatesWhenEnabling=reset
  Add : Sum
  Add1 : Sum
  Data Type Conversion : DataTypeConversion  OutDataTypeStr=single
  Data Type Conversion1 : DataTypeConversion  OutDataTypeStr=single
  Data Type Conversion2 : DataTypeConversion  OutDataTypeStr=single
  Gain : Gain  Gain=0.5
  VPER_RCenterLineC0_m : Outport
  VPER_RCenterLineC1_rad : Outport  Port=2
  VPER_RCenterLineC2_rat : Outport  Port=3
  VPER_RCenterLineC3_rat : Outport  Port=4
  wires:
  VDINR_LaneC3R_rat/1 -> Data Type Conversion2/1
  VDINR_LaneC2R_rat/1 -> Data Type Conversion1/1
  VDINR_LaneC0R_m/1 -> Add1/2, Add/2
  VPER_LaneWidth_m/1 -> Add/1
  VDINR_LaneC1R_rad/1 -> Data Type Conversion/1
  Add/1 -> Add1/1
  Add1/1 -> Gain/1
  Gain/1 -> VPER_RCenterLineC0_m/1  "VPER_RCenterLineC0_m"
  Data Type Conversion/1 -> VPER_RCenterLineC1_rad/1  "VPER_RCenterLineC1_rad"
  Data Type Conversion1/1 -> VPER_RCenterLineC2_rat/1  "VPER_RCenterLineC2_rat"
  Data Type Conversion2/1 -> VPER_RCenterLineC3_rat/1  "VPER_RCenterLineC3_rat"

== system lpr/Lane_Process/LeftLineCalculation/LR_NotAvailable ==
  Enable : EnablePort  StatesWhenEnabling=reset
  Constant : Constant  Value=1.6  OutDataTypeStr=single
  Constant1 : Constant  Value=0  OutDataTypeStr=single
  Constant2 : Constant  Value=0  OutDataTypeStr=single
  Constant3 : Constant  Value=0  OutDataTypeStr=single
  VPER_NoLeftLineC0_m : Outport
  VPER_NoLeftLineC1_rad : Outport  Port=2
  VPER_NoLeftLineC2_rat : Outport  Port=3
  VPER_NoLeftLineC3_rat : Outport  Port=4
  wires:
  Constant3/1 -> VPER_NoLeftLineC3_rat/1  "VPER_NoLeftLineC3_rat"
  Constant2/1 -> VPER_NoLeftLineC2_rat/1  "VPER_NoLeftLineC2_rat"
  Constant1/1 -> VPER_NoLeftLineC1_rad/1  "VPER_NoLeftLineC1_rad"
  Constant/1 -> VPER_NoLeftLineC0_m/1  "VPER_NoLeftLineC0_m"

== system lpr/Lane_Process/LeftLineCalculation/OnlyL_Available ==
  VDINR_LaneC0L_m : Inport
  VDINR_LaneC1L_rad : Inport  Port=2
  VDINR_LaneC2L_rat : Inport  Port=3
  VDINR_LaneC3L_rat : Inport  Port=4
  Enable : EnablePort  StatesWhenEnabling=reset
  Data Type Conversion{,1..3} (4 alike) : DataTypeConversion  OutDataTypeStr=single
  VPER_LLeftLineC0_m : Outport
  VPER_LLeftLineC1_rad : Outport  Port=2
  VPER_LLeftLineC2_rat : Outport  Port=3
  VPER_LLeftLineC3_rat : Outport  Port=4
  wires:
  Data Type Conversion/1 -> VPER_LLeftLineC1_rad/1  "VPER_LLeftLineC1_rad"
  Data Type Conversion2/1 -> VPER_LLeftLineC3_rat/1  "VPER_LLeftLineC3_rat"
  Data Type Conversion1/1 -> VPER_LLeftLineC2_rat/1  "VPER_LLeftLineC2_rat"
  Data Type Conversion3/1 -> VPER_LLeftLineC0_m/1  "VPER_LLeftLineC0_m"
  VDINR_LaneC3L_rat/1 -> Data Type Conversion2/1
  VDINR_LaneC2L_rat/1 -> Data Type Conversion1/1
  VDINR_LaneC0L_m/1 -> Data Type Conversion3/1
  VDINR_LaneC1L_rad/1 -> Data Type Conversion/1

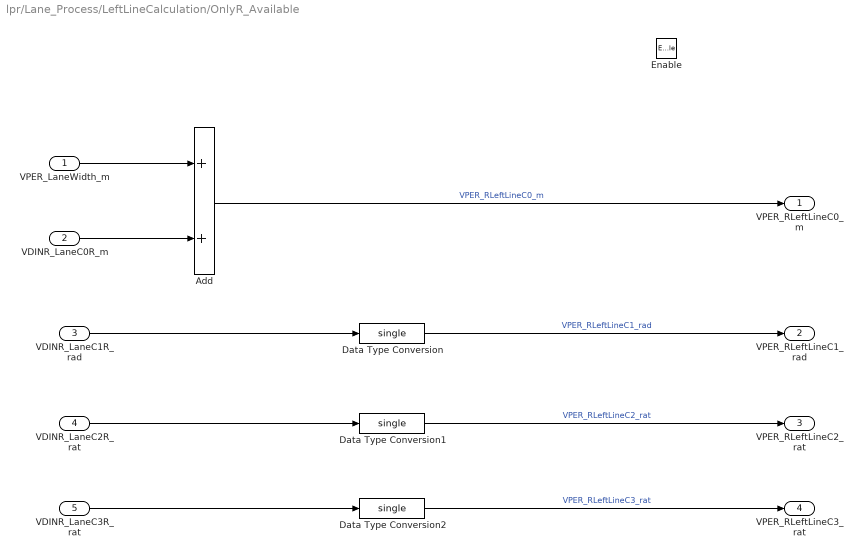
== system lpr/Lane_Process/LeftLineCalculation/OnlyR_Available ==
  VPER_LaneWidth_m : Inport
  VDINR_LaneC0R_m : Inport  Port=2
  VDINR_LaneC1R_rad : Inport  Port=3
  VDINR_LaneC2R_rat : Inport  Port=4
  VDINR_LaneC3R_rat : Inport  Port=5
  Enable : EnablePort  StatesWhenEnabling=reset
  Add : Sum
  Data Type Conversion : DataTypeConversion  OutDataTypeStr=single
  Data Type Conversion1 : DataTypeConversion  OutDataTypeStr=single
  Data Type Conversion2 : DataTypeConversion  OutDataTypeStr=single
  VPER_RLeftLineC0_m : Outport
  VPER_RLeftLineC1_rad : Outport  Port=2
  VPER_RLeftLineC2_rat : Outport  Port=3
  VPER_RLeftLineC3_rat : Outport  Port=4
  wires:
  Data Type Conversion2/1 -> VPER_RLeftLineC3_rat/1  "VPER_RLeftLineC3_rat"
  Data Type Conversion1/1 -> VPER_RLeftLineC2_rat/1  "VPER_RLeftLineC2_rat"
  Data Type Conversion/1 -> VPER_RLeftLineC1_rad/1  "VPER_RLeftLineC1_rad"
  Add/1 -> VPER_RLeftLineC0_m/1  "VPER_RLeftLineC0_m"
  VDINR_LaneC1R_rad/1 -> Data Type Conversion/1
  VPER_LaneWidth_m/1 -> Add/1
  VDINR_LaneC0R_m/1 -> Add/2
  VDINR_LaneC2R_rat/1 -> Data Type Conversion1/1
  VDINR_LaneC3R_rat/1 -> Data Type Conversion2/1

== system lpr/Lane_Process/RightLineCalculation/LR_NotAvailable ==
  Enable : EnablePort  StatesWhenEnabling=reset
  Constant : Constant  Value=-1.6  OutDataTypeStr=single
  Constant1 : Constant  Value=0  OutDataTypeStr=single
  Constant2 : Constant  Value=0  OutDataTypeStr=single
  Constant3 : Constant  Value=0  OutDataTypeStr=single
  VPER_NoRightLineC0_m : Outport
  VPER_NoRightLineC1_rad : Outport  Port=2
  VPER_NoRightLineC2_rat : Outport  Port=3
  VPER_NoRightLineC3_rat : Outport  Port=4
  wires:
  Constant/1 -> VPER_NoRightLineC0_m/1  "VPER_NoRightLineC0_m"
  Constant1/1 -> VPER_NoRightLineC1_rad/1  "VPER_NoRightLineC1_rad"
  Constant2/1 -> VPER_NoRightLineC2_rat/1  "VPER_NoRightLineC2_rat"
  Constant3/1 -> VPER_NoRightLineC3_rat/1  "VPER_NoRightLineC3_rat"

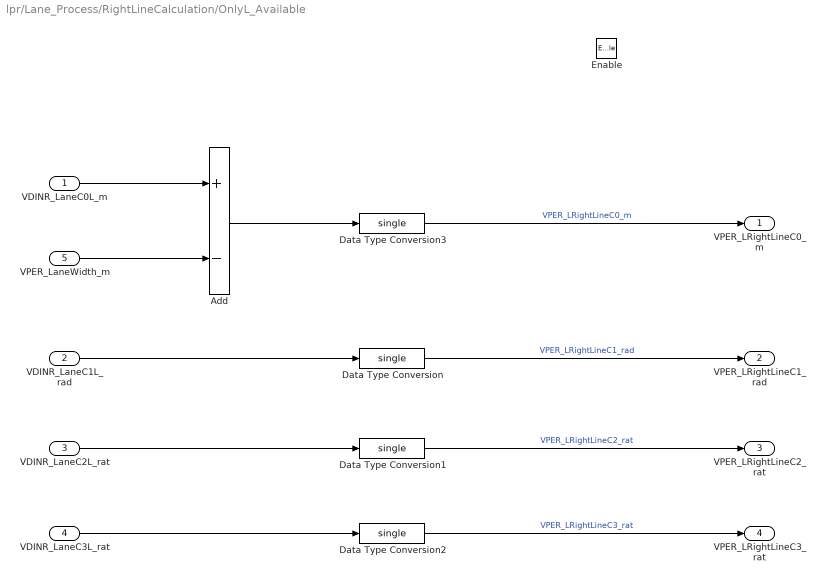
== system lpr/Lane_Process/RightLineCalculation/OnlyL_Available ==
  VDINR_LaneC0L_m : Inport
  VDINR_LaneC1L_rad : Inport  Port=2
  VDINR_LaneC2L_rat : Inport  Port=3
  VDINR_LaneC3L_rat : Inport  Port=4
  VPER_LaneWidth_m : Inport  Port=5
  Enable : EnablePort  StatesWhenEnabling=reset
  Add : Sum  Inputs=+-
  Data Type Conversion{,1..3} (4 alike) : DataTypeConversion  OutDataTypeStr=single
  VPER_LRightLineC0_m : Outport
  VPER_LRightLineC1_rad : Outport  Port=2
  VPER_LRightLineC2_rat : Outport  Port=3
  VPER_LRightLineC3_rat : Outport  Port=4
  wires:
  VDINR_LaneC1L_rad/1 -> Data Type Conversion/1
  VDINR_LaneC0L_m/1 -> Add/1
  VDINR_LaneC2L_rat/1 -> Data Type Conversion1/1
  VDINR_LaneC3L_rat/1 -> Data Type Conversion2/1
  Data Type Conversion3/1 -> VPER_LRightLineC0_m/1  "VPER_LRightLineC0_m"
  Data Type Conversion1/1 -> VPER_LRightLineC2_rat/1  "VPER_LRightLineC2_rat"
  Data Type Conversion2/1 -> VPER_LRightLineC3_rat/1  "VPER_LRightLineC3_rat"
  Data Type Conversion/1 -> VPER_LRightLineC1_rad/1  "VPER_LRightLineC1_rad"
  VPER_LaneWidth_m/1 -> Add/2
  Add/1 -> Data Type Conversion3/1

== system lpr/Lane_Process/RightLineCalculation/OnlyR_Available ==
  VDINR_LaneC0R_m : Inport
  VDINR_LaneC1R_rad : Inport  Port=2
  VDINR_LaneC2R_rat : Inport  Port=3
  VDINR_LaneC3R_rat : Inport  Port=4
  Enable : EnablePort  StatesWhenEnabling=reset
  Data Type Conversion{,1..3} (4 alike) : DataTypeConversion  OutDataTypeStr=single
  VPER_RRightLineC0_m : Outport
  VPER_RRightLineC1_rad : Outport  Port=2
  VPER_RRightLineC2_rat : Outport  Port=3
  VPER_RRightLineC3_rat : Outport  Port=4
  wires:
  VDINR_LaneC3R_rat/1 -> Data Type Conversion2/1
  VDINR_LaneC2R_rat/1 -> Data Type Conversion1/1
  VDINR_LaneC1R_rad/1 -> Data Type Conversion/1
  VDINR_LaneC0R_m/1 -> Data Type Conversion3/1
  Data Type Conversion/1 -> VPER_RRightLineC1_rad/1  "VPER_RRightLineC1_rad"
  Data Type Conversion1/1 -> VPER_RRightLineC2_rat/1  "VPER_RRightLineC2_rat"
  Data Type Conversion2/1 -> VPER_RRightLineC3_rat/1  "VPER_RRightLineC3_rat"
  Data Type Conversion3/1 -> VPER_RRightLineC0_m/1  "VPER_RRightLineC0_m"

== stateflow chart Lane_Process/CenterLineCalculation/Lane_status ==
  (default) -> (junction 12)
  (junction 12) -> (junction 13) [order 1] : [VPER_LeftLaneAvail_fig && VPER_RightLaneAvail_fig]
  (junction 12) -> (junction 14) [order 2]
  (junction 13) -> (junction 21) : {SWCase=1;
      | LR_avail=TRUE;
      | R_avail=FALSE;
      | L_avail=FALSE;
      | NO_avail=FALSE;}
  (junction 14) -> (junction 15) [order 1] : [!VPER_LeftLaneAvail_fig && VPER_RightLaneAvail_fig]
  (junction 14) -> (junction 16) [order 2]
  (junction 15) -> (junction 20) : {SWCase=2;
      | LR_avail=FALSE;
      | R_avail=TRUE;
      | L_avail=FALSE;
      | NO_avail=FALSE;}
  (junction 16) -> (junction 17) [order 1] : [VPER_LeftLaneAvail_fig && !VPER_RightLaneAvail_fig]
  (junction 16) -> (junction 18) [order 2] : {SWCase=4;
      | LR_avail=FALSE;
      | R_avail=FALSE;
      | L_avail=FALSE;
      | NO_avail=TRUE;}
  (junction 17) -> (junction 19) : {SWCase=3;
      | LR_avail=FALSE;
      | R_avail=FALSE;
      | L_avail=TRUE;
      | NO_avail=FALSE;}
  (junction 19) -> (junction 18)
  (junction 20) -> (junction 19)
  (junction 21) -> (junction 20)
  data: VPER_LeftLaneAvail_fig input double; VPER_RightLaneAvail_fig input double; SWCase output single; LR_avail output boolean; R_avail output boolean; L_avail output boolean; NO_avail output boolean; TRUE parameter double; FALSE parameter double

== stateflow chart Lane_Process/LeftLineCalculation/Lane_status ==
  (default) -> (junction 45)
  (junction 45) -> (junction 46) [order 1] : [VPER_LeftLaneAvail_fig]
  (junction 45) -> (junction 47) [order 2]
  (junction 46) -> (junction 51) : {SWCase=1;
      | R_avail=FALSE;
      | L_avail=TRUE;
      | NO_avail=FALSE;}
  (junction 47) -> (junction 48) [order 2] : [!VPER_LeftLaneAvail_fig && VPER_RightLaneAvail_fig]
  (junction 47) -> (junction 49) [order 1] : {SWCase=3;
      | R_avail=FALSE;
      | L_avail=FALSE;
      | NO_avail=TRUE;}
  (junction 48) -> (junction 50) : {SWCase=2;
      | R_avail=TRUE;
      | L_avail=FALSE;
      | NO_avail=FALSE;}
  (junction 50) -> (junction 49)
  (junction 51) -> (junction 50)
  data: VPER_LeftLaneAvail_fig input double; VPER_RightLaneAvail_fig input double; SWCase output single; R_avail output boolean; L_avail output boolean; NO_avail output boolean; TRUE parameter double; FALSE parameter double

== stateflow chart Lane_Process/RightLineCalculation/Lane_status ==
  (default) -> (junction 71)
  (junction 71) -> (junction 72) [order 1] : [VPER_RightLaneAvail_fig]
  (junction 71) -> (junction 73) [order 2]
  (junction 72) -> (junction 77) : {SWCase=1;
      | R_avail=TRUE;
      | L_avail=FALSE;
      | NO_avail=FALSE;}
  (junction 73) -> (junction 74) [order 2] : [!VPER_RightLaneAvail_fig && VPER_LeftLaneAvail_fig]
  (junction 73) -> (junction 75) [order 1] : {SWCase=3;
      | R_avail=FALSE;
      | L_avail=FALSE;
      | NO_avail=TRUE;}
  (junction 74) -> (junction 76) : {SWCase=2;
      | R_avail=FALSE;
      | L_avail=TRUE;
      | NO_avail=FALSE;}
  (junction 76) -> (junction 75)
  (junction 77) -> (junction 76)
  data: VPER_LeftLaneAvail_fig input double; VPER_RightLaneAvail_fig input double; SWCase output single; R_avail output boolean; L_avail output boolean; NO_avail output boolean; TRUE parameter double; FALSE parameter double
